simulink model "picam_LaneDeparture"  (R2017a)
settings: Solver=FixedStepAuto  StartTime=0.0  StopTime=inf  FixedStep=1/40  RelTol=1e-3  EnableMultiTasking=on
libraries: visionsinks x1, dspvision x1, embdlinuxlib x1
settings Model: Creator=ChiChaChai  LastModifiedBy=Vincent
settings SolverCC: PositivePriorityOrder=on  AutoInsertRateTranBlk=on
settings OptimizationCC: UseFloatMulNetSlope=on  PassReuseOutputArgsThreshold=0  EfficientFloat2IntCast=on  LifeSpan=1  MaxStackSize=64
settings DebuggingCC: ParameterTunabilityLossMsg=error
settings HardwareCC: ProdBitPerPointer=32  ProdBitPerSizeT=32  ProdBitPerPtrDiffT=32  ProdLargestAtomicInteger=Long  ProdLargestAtomicFloat=Double  ProdWordSize=32  ProdHWDeviceType=ARM Compatible->ARM Cortex
settings ModelReferenceCC: PropagateVarSize=During execution
settings SFSimCC: MATLABDynamicMemAlloc=off
settings RTWCC: SystemTargetFile=ert.tlc  HardwareBoard=Raspberry Pi  TLCOptions="-aInlineSetEventsForThisBaseRateFcn=TLC_FALSE -aSuppressMultiTaskScheduler=TLC_FALSE  -aRateBasedStepFcn=0"  TemplateMakefile=ert_default_tmf  Description=Embedded Coder  GenerateReport=on  Toolchain=GNU GCC Raspberry Pi  LaunchReport=on
settings CodeAppCC: ForceParamTrailComments=on  OperatorAnnotations=on  MATLABSourceComments=on
settings ERTTargetCC: CombineSignalStateStructs=on  ERTCustomFileBanners=off  SupportContinuousTime=on  SupportNonInlinedSFcns=on  RemoveResetFunc=off  SupportVariableSizeSignals=on  ModelStepFunctionPrototypeControlCompliant=off  ExtMode=on  ExtModeMexArgs='192.168.1.228' 0 17725  ERTFilePackagingFormat=CompactWithDataFile

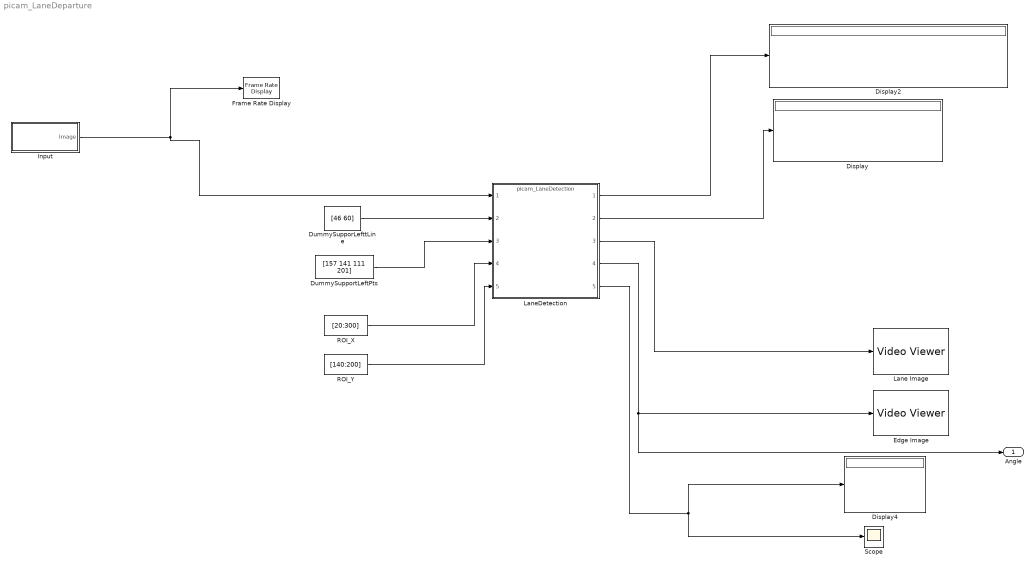
== system picam_LaneDeparture ==
  Display : Display
  Display2 : Display
  Display4 : Display
  DummySupporLefttLine : Constant  Value=[46 60]  VectorParams1D=off  OutDataTypeStr=double
  DummySupportLeftPts : Constant  Value=[157 141 111 201]  OutDataTypeStr=double
  Edge Image : VideoViewer  FigPos=[958 673 304 248]
  Frame Rate Display : visionsinks/Frame Rate Display  UpdateRate=10
      settings: SourceProductName=Computer Vision System Toolbox  SourceProductBaseCode=VP
  "Input " : Subsystem
  Lane Image : VideoViewer  FigPos=[765 746 343 246]
  LaneDetection : ModelReference  ModelNameDialog=picam_LaneDetection.slx  SimulationMode=Normal  ModelReferenceVersion=1.331
  ROI_X : Constant  Value=[20:300]  LockScale=on
  ROI_Y : Constant  Value=[140:200]  LockScale=on
  Scope : Scope
  Angle : Outport  SampleTime=1/40
  wires:
  LaneDetection/3 -> Lane Image/1
  LaneDetection/4 -> Angle/1, Edge Image/1
  LaneDetection/2 -> Display/1
  DummySupporLefttLine/1 -> LaneDetection/2
  LaneDetection/5 -> Display4/1, Scope/1
  LaneDetection/1 -> Display2/1
  "Input "/1(Image) -> LaneDetection/1, Frame Rate Display/1
  DummySupportLeftPts/1 -> LaneDetection/3
  ROI_X/1 -> LaneDetection/4
  ROI_Y/1 -> LaneDetection/5

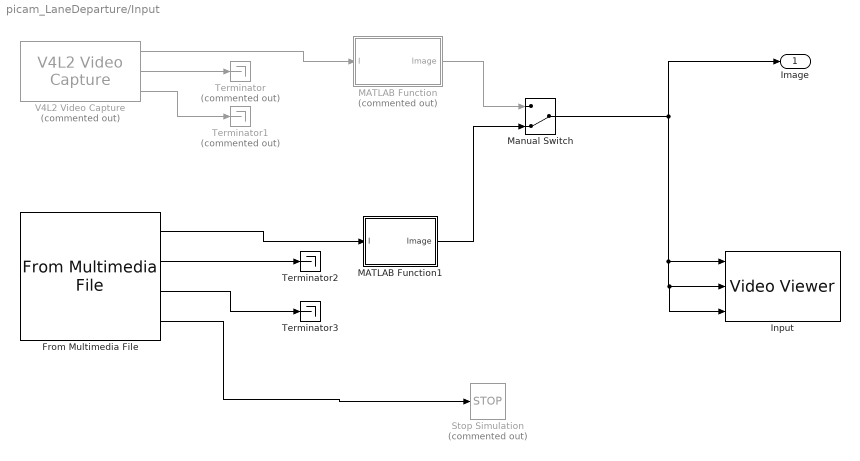
== system picam_LaneDeparture/Input  ==
  From Multimedia File : dspvision/From Multimedia File  inputFilename=/Users/Vincent/Documents/GitHub/AMBD/testing_src/video3.mp4  loop=on  numPlays=inf  outputStreams=Video only  videoDataType=uint8  audioDataType=int16  inheritSampleTime=off  userDefinedSampleTime=1/20  noAudioOutput=off  isIntensityVideo=off  fourcc=YCbCr 4:2:2  colorVideoFormat=One multidimensional signal  outputEOF=on  dataOrg=Column-major  audioFrameSize=1024  computeAudioFrameSize=off  outSamplingMode=Sample based
      settings: SourceProductBaseCode=VP
  Input : VideoViewer  imagePorts=separate color signals  FigPos=[29 956 1279 247]
  MATLAB Function : MATLAB Function  Commented=on  TreatAsAtomicUnit=on
  MATLAB Function1 : MATLAB Function  TreatAsAtomicUnit=on
  Manual Switch : ManualSwitch  CurrentSetting=0
  Stop Simulation : Stop  Commented=on
  Terminator : Terminator  Commented=on
  Terminator1 : Terminator  Commented=on
  Terminator2 : Terminator
  Terminator3 : Terminator
  V4L2 Video Capture : embdlinuxlib/V4L2 Video Capture  Commented=on  m_devName='/dev/video0'  roi=[0, 0, 640, 480]  imSizeSelection=320x240  imSize=[640, 480]  pixelFormat=YCbCr 4:2:2  pixelOrder=Planar  sampleTime=1/50  simOutput=Colorbars  blockPlatform=Raspberry Pi
  Image : Outport
  wires:
  V4L2 Video Capture/2 -> Terminator/1
  V4L2 Video Capture/3 -> Terminator1/1
  V4L2 Video Capture/1 -> MATLAB Function/1(I)
  From Multimedia File/2 -> Terminator2/1
  From Multimedia File/3 -> Terminator3/1
  From Multimedia File/1 -> MATLAB Function1/1(I)
  From Multimedia File/4 -> Stop Simulation/1
  MATLAB Function/1(Image) -> Manual Switch/1
  MATLAB Function1/1(Image) -> Manual Switch/2
  Manual Switch/1 -> Input/3, Input/2, Input/1, Image/1

== matlab function picam_LaneDeparture/Input /MATLAB Function1 ==
  data: I input; Image output
function Image = Flip(I)

Image = imrotate(I,180,'bilinear');

== matlab function picam_LaneDeparture/Input /MATLAB Function ==
  data: I input; Image output
function Image = FlipAndRotate(I)
Image = imrotate(I,90,'bilinear');
Image = flip(Image,2);
